simulink model "errorbase_control"  (R2019b)
settings: Solver=FixedStepAuto  StartTime=0.0  StopTime=inf  RelTol=1e-3  EnableMultiTasking=on
libraries: arduinolib x4
settings Model: SILPILModeSetting=veronly  ExtModeTrigDuration=2  Creator=Agc  LastModifiedBy=Agc
settings OptimizationCC: EnhancedBackFolding=on  PassReuseOutputArgsAs=Individual arguments  ZeroExternalMemoryAtStartup=off  ZeroInternalMemoryAtStartup=off  MaxStackSize=64  OptimizeBlockOrder=speed  DifferentSizesBufferReuse=on  OptimizationCustomize=off  EfficientTunableParamExpr=on
settings DebuggingCC: ParameterTunabilityLossMsg=error
settings HardwareCC: ProdBitPerInt=16  ProdBitPerPointer=16  ProdBitPerSizeT=16  ProdBitPerPtrDiffT=16  ProdLargestAtomicFloat=None  ProdWordSize=8  ProdHWDeviceType=Atmel->AVR
settings SFSimCC: MATLABDynamicMemAlloc=off
settings RTWCC: SystemTargetFile=ert.tlc  HardwareBoard=Arduino Mega 2560  TLCOptions=-aInlineSetEventsForThisBaseRateFcn=TLC_FALSE -aSuppressMultiTaskScheduler=TLC_FALSE -aRateBasedStepFcn=1  TemplateMakefile=ert_default_tmf  GenerateReport=on  Toolchain=Arduino AVR  BuildConfiguration=Faster Runs  IncludeHyperlinkInReport=on  LaunchReport=on  GenerateTraceInfo=on  GenerateTraceReport=on  GenerateTraceReportSl=on  GenerateTraceReportSf=on  GenerateTraceReportEml=on
settings CodeAppCC: ForceParamTrailComments=on  IgnoreCustomStorageClasses=off  OperatorAnnotations=on  SimulinkDataObjDesc=on  SFDataObjDesc=on  InsertBlockDesc=on
settings ERTTargetCC: SupportContinuousTime=on  SupportVariableSizeSignals=on  ExtModeStaticAllocSize=2048

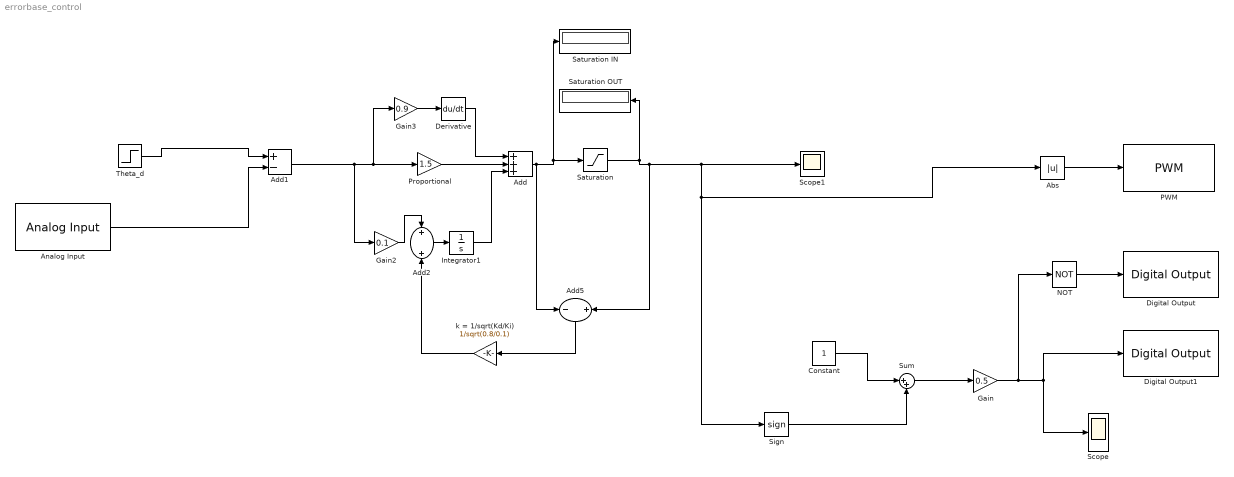
== system errorbase_control ==
  Abs : Abs
  Add : Sum  Inputs=+++
  Add1 : Sum  Inputs=+-
  Add2 : Sum
  Add5 : Sum  Inputs=-+
  Analog Input : arduinolib/Analog Input  pinNumber=0  ReadResultsOnly=off  ConversionTriggerSource=Software  ExternalTriggerType=uint32(0)  OutputDataType=uint16  EnableConversionCompleteNotify=off  EnableOuputStatus=off  SampleTime=-1  blockPlatform=arduino
  Constant : Constant
  Derivative : Derivative
  Digital Output : arduinolib/Digital Output  pinNumber=11  blockPlatform=arduino
  Digital Output1 : arduinolib/Digital Output  pinNumber=12  blockPlatform=arduino
  Gain : Gain  Gain=0.5
  Gain2 : Gain  Gain=0.1
  Gain3 : Gain  Gain=0.9
  Integrator1 : Integrator
  NOT : Logic  Operator=NOT  IconShape=distinctive  AllPortsSameDT=off  OutDataTypeStr=boolean
  PWM : arduinolib/PWM  pinNumber=13  EnableInputFrequency=off  InitialFrequency=2000  InitialDutyCycle=0  NotificationType=None  blockPlatform=arduino
  Proportional : Gain  Gain=1.5
  Saturation : Saturate  UpperLimit=130  LowerLimit=-130
  Saturation IN : Display
  Saturation OUT : Display
  Scope : Scope
  Scope1 : Scope
  Sign : Signum
  Sum : Sum  Inputs=|++
  Theta_d : Step  After=95  SampleTime=0
  k = 1/sqrt(Kd/Ki) : Gain  Gain=1/sqrt(0.8/0.1)
  wires:
  NOT/1 -> Digital Output/1
  Constant/1 -> Sum/1
  Sum/1 -> Gain/1
  Gain/1 -> NOT/1, Digital Output1/1, Scope/1
  Sign/1 -> Sum/2
  Integrator1/1 -> Add/3
  Gain3/1 -> Derivative/1
  Proportional/1 -> Add/2
  Derivative/1 -> Add/1
  Analog Input/1 -> Add1/2
  Abs/1 -> PWM/1
  Theta_d/1 -> Add1/1
  Gain2/1 -> Add2/1
  k = 1/sqrt(Kd/Ki)/1 -> Add2/2
  Add5/1 -> k = 1/sqrt(Kd/Ki)/1
  Saturation/1 -> Add5/2, Abs/1, Sign/1, Scope1/1, Saturation OUT/1
  Add2/1 -> Integrator1/1
  Add/1 -> Add5/1, Saturation IN/1, Saturation/1
  Add1/1 -> Gain3/1, Proportional/1, Gain2/1
